simulink model "arduino_lab_R2016a"  (R2016a)
settings: Solver=VariableStepAuto  StartTime=0.0  StopTime=500  RelTol=1e-3
StartFcn:
  | clear all
libraries: simulink x2, realtime_pacer_lib x1
settings Model: Creator=johnh  LastModifiedBy=johnh

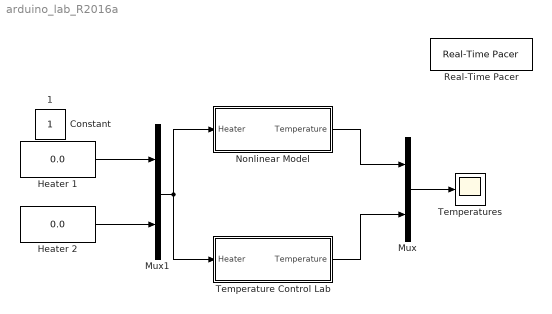
== system arduino_lab_R2016a ==
  Heater 1 : simulink/Math Operations/Slider Gain  gain=0.0  low=0  high=100
  Heater 2 : simulink/Math Operations/Slider Gain  gain=0.0  low=0  high=100
  Mux : Mux  Inputs=2
  Mux1 : Mux  Inputs=2
  Nonlinear Model : Subsystem
  Real-Time Pacer : realtime_pacer_lib/Real-Time Pacer  simTimePerRealTime=1
  Temperature Control Lab : Subsystem
  Temperatures : Scope
  1 : Constant  IOType=siggen
  Constant : Constant  IOType=siggen
  wires:
  Mux/1 -> Temperatures/1
  Nonlinear Model/1(Temperature) -> Mux/1
  Temperature Control Lab/1(Temperature) -> Mux/2
  Heater 1/1 -> Mux1/1
  Heater 2/1 -> Mux1/2
  Mux1/1 -> Temperature Control Lab/1(Heater), Nonlinear Model/1(Heater)

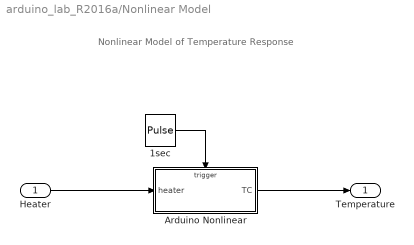
== system arduino_lab_R2016a/Nonlinear Model ==
  note: Nonlinear Model of Temperature Response
  Heater : Inport
  1sec : DiscretePulseGenerator  PulseType=Time based  Period=1  PulseWidth=50
  Arduino Nonlinear : Subsystem  TreatAsAtomicUnit=on
  Temperature : Outport
  wires:
  1sec/1 -> Arduino Nonlinear/Trigger
  Arduino Nonlinear/1(TC) -> Temperature/1
  Heater/1 -> Arduino Nonlinear/1(heater)

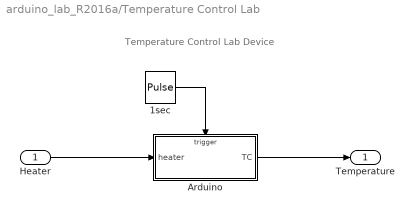
== system arduino_lab_R2016a/Temperature Control Lab ==
  note: Temperature Control Lab Device
  Heater : Inport
  1sec : DiscretePulseGenerator  PulseType=Time based  Period=1  PulseWidth=50
  Arduino : Subsystem  TreatAsAtomicUnit=on
  Temperature : Outport
  wires:
  1sec/1 -> Arduino/Trigger
  Arduino/1(TC) -> Temperature/1
  Heater/1 -> Arduino/1(heater)

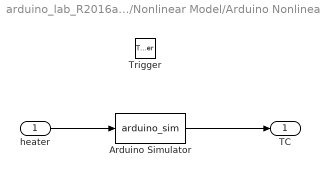
== system arduino_lab_R2016a/Nonlinear Model/Arduino Nonlinear ==
  heater : Inport
  Trigger : TriggerPort  VariantControl=Variant
  Arduino Simulator : MATLABFcn  MATLABFcn=arduino_sim
  TC : Outport  InitialOutput=23
  wires:
  heater/1 -> Arduino Simulator/1
  Arduino Simulator/1 -> TC/1

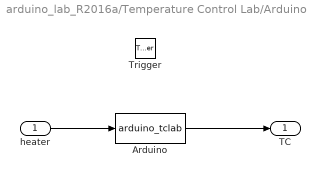
== system arduino_lab_R2016a/Temperature Control Lab/Arduino ==
  heater : Inport  LatchByDelayingOutsideSignal=on
  Trigger : TriggerPort  VariantControl=Variant
  Arduino : MATLABFcn  MATLABFcn=arduino_tclab
  TC : Outport  InitialOutput=23
  wires:
  heater/1 -> Arduino/1
  Arduino/1 -> TC/1
